simulink model "SumGain"  (R2021a)
settings: Solver=VariableStepAuto  StartTime=0.0  StopTime=10.0  RelTol=1e-3
settings Model: Creator=20204920  LastModifiedBy=20204920
settings OptimizationCC: ZeroExternalMemoryAtStartup=off  ZeroInternalMemoryAtStartup=off
settings RTWCC: TargetLang=C++
settings GRTTargetCC: TargetLangStandard=C++03 (ISO)  CodeInterfacePackaging=C++ class

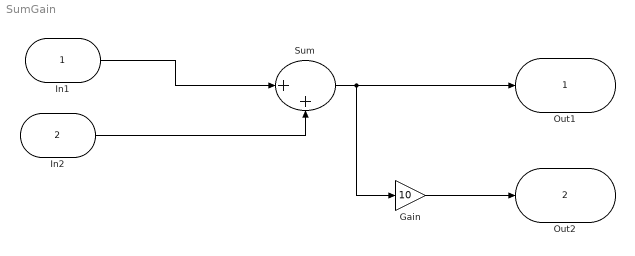
== system SumGain ==
  In1 : Inport  OutDataTypeStr=int32
  In2 : Inport  Port=2  OutDataTypeStr=int32
  Gain : Gain  Gain=10
  Sum : Sum  Inputs=|++
  Out1 : Outport  OutDataTypeStr=int32
  Out2 : Outport  Port=2  OutDataTypeStr=int32
  wires:
  In1/1 -> Sum/1
  In2/1 -> Sum/2
  Sum/1 -> Gain/1, Out1/1
  Gain/1 -> Out2/1
